simulink model "Control_Modelo"  (R2020b)
settings: Solver=VariableStepAuto  StartTime=0.0  StopTime=inf  RelTol=1e-3
values from neighbouring files (symbols this model uses):
  kd = kp/500    (= 0.0036)    [PID.m]
  ki = 0    [PID.m]
  kp = 1.8    [PID.m]
undefined symbols (not defined in the file or in its folder): a, b, serial
libraries: instrumentlib x2, pid_lib x1
settings Model: Creator=Dell  LastModifiedBy=Dell

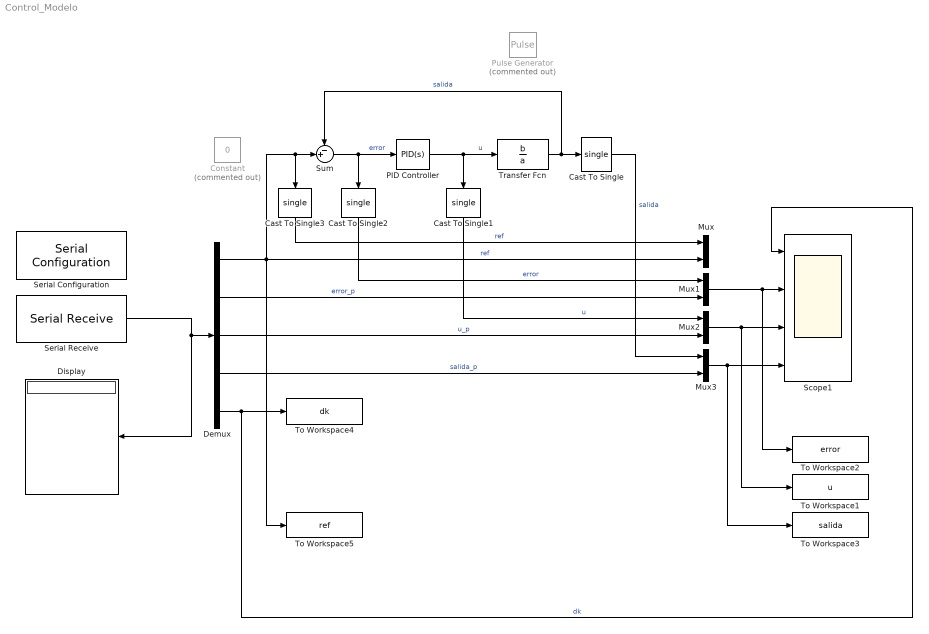
== system Control_Modelo ==
  Cast To Single{,1..3} (4 alike) : DataTypeConversion  OutDataTypeStr=single
  Constant : Constant  Commented=on  Value=0
  Demux : Demux  Outputs=5
  Display : Display
  Mux{,1..3} (4 alike) : Mux  Inputs=2
  PID Controller : pid_lib/PID Controller  Controller=PID  Form=Parallel  TimeDomain=Continuous-time  UseExternalTs=off  SampleTime=-1  IntegratorMethod=Forward Euler  FilterMethod=Forward Euler  ControllerParametersSource=internal  P=kp  I=ki  D=kd  UseFilter=on  N=100  TunerSelectOption=Transfer Function Based (PID Tuner App)  InitialConditionSource=internal  InitialConditionForIntegrator=0  InitialConditionForFilter=0  DifferentiatorICPrevScaledInput=0  ExternalReset=none  TrackingMode=off  Kt=1  LimitOutput=off  SatLimitsSource=internal  UpperSaturationLimit=inf  LowerSaturationLimit=-inf  LinearizeAsGain=on  AntiWindupMode=none  Kb=1  POutMin=[]  POutMax=[]  IOutMin=[]  IOutMax=[]  DOutMin=[]  DOutMax=[]  NOutMin=[]  NOutMax=[]  SumOutMin=[]  SumOutMax=[]  SaturationOutMin=[]  SaturationOutMax=[]  PParamMin=[]  PParamMax=[]  IParamMin=[]  IParamMax=[]  DParamMin=[]  DParamMax=[]  NParamMin=[]  NParamMax=[]  KbParamMin=[]  KbParamMax=[]  KtParamMin=[]  KtParamMax=[]  KbOutMin=[]  KbOutMax=[]  KtOutMin=[]  KtOutMax=[]  IntegratorOutMin=[]  IntegratorOutMax=[]  FilterOutMin=[]  FilterOutMax=[]  SumI1OutMin=[]  SumI1OutMax=[]  SumI2OutMin=[]  SumI2OutMax=[]  SumI3OutMin=[]  SumI3OutMax=[]  SumI4OutMin=[]  SumI4OutMax=[]  SumDOutMin=[]  SumDOutMax=[]  DifferentiatorOutMin=[]  DifferentiatorOutMax=[]  FilterDiffOutCoefMin=[]  FilterDiffOutCoefMax=[]  ReciprocalOutMin=[]  ReciprocalOutMax=[]  SumDenOutMin=[]  SumDenOutMax=[]  SumNumOutMin=[]  SumNumOutMax=[]  DivideOutMin=[]  DivideOutMax=[]  UdiffTsProdOutMin=[]  UdiffTsProdOutMax=[]  NTsProdOutMin=[]  NTsProdOutMax=[]  UintegralTsProdOutMin=[]  UintegralTsProdOutMax=[]  UngainTsProdOutMin=[]  UngainTsProdOutMax=[]  IntegratorContinuousStateAttributes=''  IntegratorStateMustResolveToSignalObject=off  IntegratorRTWStateStorageClass=Auto  FilterContinuousStateAttributes=''  FilterStateMustResolveToSignalObject=off  FilterRTWStateStorageClass=Auto  ParallelPVariant=InternalParameters  IdealPVariant=Disabled  IVariant=InternalParameters  DVariant=InternalParameters  IntegratorVariant=Continuous  SatVariant=Disabled  AWVariant=Passthrough  PCopyVariant=Disabled  TRVariant=Disabled  FdbkBlocksVariant=Forward  IdealPFdbkVariant=Disabled  SatFdbkVariant=Disabled  DerivativeFilterVariant=ContFilter  NVariant=InternalParameters  NCopyVariant=Disabled  FilterICVariant=InternalICsFilter  IntegratorICVariant=InternalICs  ExternalResetVariant=Disabled  TRSumVariant=Passthrough  SumFdbkVariant=Disabled  SumVariant=Sum_PID  TsampFilterVariant=InternalTs  TsampNgainVariant=Passthrough  TsampIntegralVariant=Passthrough  ExternalSaturationOutDataTypeStr=Inherit: Same as second input
  Pulse Generator : DiscretePulseGenerator  Commented=on  PulseType=Time based  Amplitude=15  Period=1000  PulseWidth=0.1  PhaseDelay=20
  Scope1 : Scope  NumInputPorts=4
  Serial Configuration : instrumentlib/Serial Configuration  Priority=-200000  ComPortMenu=COM10  ComPort=COM10  ObjConstructor=serial('COM10');  BaudRate=115200  DataBits=8  Parity=none  StopBits=1  FlowControl=none  Timeout=10  ByteOrder=LittleEndian
  Serial Receive : instrumentlib/Serial Receive  Priority=1  ComPortMenu=COM10  ComPort=COM10  ObjConstructor=serial('COM10');  Header=abcd  Terminator=<none>  DataSize="[5  1]"  DataType=single  EnableBlockingMode=on  ActionDataUnavailable=Output last received value  CustomValue=0  SampleTime=0.02
  Sum : Sum  Inputs=-+|
  To Workspace1 : ToWorkspace  VariableName=u  SampleTime=-1
      settings: Save2DSignal=2-D array (concatenate along first dimension)
  To Workspace2 : ToWorkspace  VariableName=error  SampleTime=-1
      settings: Save2DSignal=2-D array (concatenate along first dimension)
  To Workspace3 : ToWorkspace  VariableName=salida  SampleTime=-1
      settings: Save2DSignal=2-D array (concatenate along first dimension)
  To Workspace4 : ToWorkspace  VariableName=dk  SampleTime=-1
      settings: Save2DSignal=2-D array (concatenate along first dimension)
  To Workspace5 : ToWorkspace  VariableName=ref  SampleTime=-1
      settings: Save2DSignal=2-D array (concatenate along first dimension)
  Transfer Fcn : TransferFcn  Numerator=b  Denominator=a
  wires:
  PID Controller/1 -> Cast To Single1/1, Transfer Fcn/1  "u"
  Sum/1 -> PID Controller/1, Cast To Single2/1  "error"
  Transfer Fcn/1 -> Sum/1, Cast To Single/1  "salida"
  Demux/1 -> To Workspace5/1, Sum/2, Cast To Single3/1, Mux/2  "ref"
  Mux1/1 -> To Workspace2/1, Scope1/2
  Mux2/1 -> To Workspace1/1, Scope1/3
  Mux3/1 -> To Workspace3/1, Scope1/4
  Demux/2 -> Mux1/2  "error_p"
  Demux/3 -> Mux2/2  "u_p"
  Demux/4 -> Mux3/2  "salida_p"
  Serial Receive/1 -> Display/1, Demux/1
  Cast To Single/1 -> Mux3/1  "salida"
  Cast To Single1/1 -> Mux2/1  "u"
  Cast To Single2/1 -> Mux1/1  "error"
  Cast To Single3/1 -> Mux/1  "ref"
  Demux/5 -> To Workspace4/1, Scope1/1  "dk"
